simulink model "q3a3576a"  (Simulink 7.7)
settings: Solver=ode45  StartTime=0.0  StopTime=10.0  RelTol=1e-3
libraries: simulink x1
settings Model: Creator=Owner  LastModifiedBy=Owner

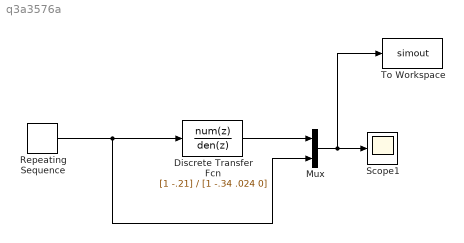
== system q3a3576a ==
  Discrete Transfer Fcn : DiscreteTransferFcn  Numerator=[1 -.21]  Denominator=[1 -.34 .024 0]
  Mux : Mux  Inputs=2
  Repeating Sequence : simulink/Sources/Repeating Sequence  SystemSampleTime=-1  rep_seq_t=[0:.002:1]  rep_seq_y=[.21.^[1:1:501]]
  Scope1 : Scope
      settings: TimeRange=10  YMin=0  YMax=0.25
  To Workspace : ToWorkspace  VariableName=simout  SampleTime=-1  SaveFormat=Structure
  wires:
  Repeating Sequence/1 -> Discrete Transfer Fcn/1, Mux/2
  Discrete Transfer Fcn/1 -> Mux/1
  Mux/1 -> Scope1/1, To Workspace/1
